simulink model "NDT_Localization"  (R2022a)
settings: Solver=FixedStepAuto  StartTime=0.0  StopTime=10.0  RelTol=1e-3
model workspace (MAT data in the model file):
  SL_ROS_VariableLengthArrays_MaxSizes : object (value not decoded)
undefined symbols (not defined in the file or in its folder): null
libraries: ros2lib x9, robotlib x8, simulink x1
(part 12 of 12)

== matlab function NDT_Localization/observation_callback/check_localizer/If Action Subsystem/register_measurement_impl/If Action Subsystem/If Action Subsystem/solve/If Action Subsystem1/For Iterator Subsystem/compute_next_step/If Action Subsystem1/psi_t/initial_objective_function/For Iterator Subsystem/gradient_jaco/gradient_col ==
  data: index input; gradient input; y output
function y = fcn(index,gradient)

y = gradient(:,index);

== matlab function NDT_Localization/observation_callback/check_localizer/If Action Subsystem/register_measurement_impl/If Action Subsystem/If Action Subsystem/solve/If Action Subsystem1/For Iterator Subsystem/compute_next_step/If Action Subsystem1/psi_t/initial_objective_function/For Iterator Subsystem/gradient_jaco/jaco_add ==
  data: jacobian input; jacobian output; index input; num input
function jacobian = fcn(jacobian,index,num)

jacobian(index) = jacobian(index)+num;

== matlab function NDT_Localization/observation_callback/check_localizer/If Action Subsystem/register_measurement_impl/If Action Subsystem/If Action Subsystem/solve/If Action Subsystem1/For Iterator Subsystem/compute_next_step/If Action Subsystem1/psi_t/initial_objective_function/angle_params/MATLAB Function ==
  data: x output; u input; y output; z output
function [x,y,z] = fcn(u)
x = u(3);
y = u(4);
z = u(5);

== matlab function NDT_Localization/observation_callback/check_localizer/If Action Subsystem/register_measurement_impl/If Action Subsystem/If Action Subsystem/solve/If Action Subsystem1/For Iterator Subsystem/compute_next_step/If Action Subsystem1/psi_t/initial_objective_function/gradient_angle/ga_a ==
  data: x input; out output; y input; z input
function out = fcn(x, y, z)
out = zeros(1,3); 
out(1) = x;
out(2) = y;
out(3) = z;

== matlab function NDT_Localization/observation_callback/check_localizer/If Action Subsystem/register_measurement_impl/If Action Subsystem/If Action Subsystem/solve/If Action Subsystem1/For Iterator Subsystem/compute_next_step/If Action Subsystem1/psi_t/initial_objective_function/gradient_angle/ga_b ==
  data: x input; out output; y input; z input
function out = fcn(x, y, z)
out = zeros(1,3); 
out(1) = x;
out(2) = y;
out(3) = z;

== matlab function NDT_Localization/observation_callback/check_localizer/If Action Subsystem/register_measurement_impl/If Action Subsystem/If Action Subsystem/solve/If Action Subsystem1/For Iterator Subsystem/compute_next_step/If Action Subsystem1/psi_t/initial_objective_function/gradient_angle/ga_c ==
  data: x input; out output; y input; z input
function out = fcn(x, y, z)
out = zeros(1,3); 
out(1) = x;
out(2) = y;
out(3) = z;

== matlab function NDT_Localization/observation_callback/check_localizer/If Action Subsystem/register_measurement_impl/If Action Subsystem/If Action Subsystem/solve/If Action Subsystem1/For Iterator Subsystem/compute_next_step/If Action Subsystem1/psi_t/initial_objective_function/gradient_angle/ga_d ==
  data: x input; out output; y input; z input
function out = fcn(x, y, z)
out = zeros(1,3); 
out(1) = x;
out(2) = y;
out(3) = z;

== matlab function NDT_Localization/observation_callback/check_localizer/If Action Subsystem/register_measurement_impl/If Action Subsystem/If Action Subsystem/solve/If Action Subsystem1/For Iterator Subsystem/compute_next_step/If Action Subsystem1/psi_t/initial_objective_function/gradient_angle/ga_e ==
  data: x input; out output; y input; z input
function out = fcn(x, y, z)
out = zeros(1,3); 
out(1) = x;
out(2) = y;
out(3) = z;

== matlab function NDT_Localization/observation_callback/check_localizer/If Action Subsystem/register_measurement_impl/If Action Subsystem/If Action Subsystem/solve/If Action Subsystem1/For Iterator Subsystem/compute_next_step/If Action Subsystem1/psi_t/initial_objective_function/gradient_angle/ga_f ==
  data: x input; out output; y input; z input
function out = fcn(x, y, z)
out = zeros(1,3); 
out(1) = x;
out(2) = y;
out(3) = z;

== matlab function NDT_Localization/observation_callback/check_localizer/If Action Subsystem/register_measurement_impl/If Action Subsystem/If Action Subsystem/solve/point_hessian ==
  data: hessian output; ha_a2 input; ha_a3 input; ha_b2 input; ha_b3 input; ha_c2 input; ha_c3 input; ha_d1 input; ha_d2 input; ha_d3 input; ha_e1 input; ha_e2 input; ha_e3 input; ha_f1 input; ha_f2 input; ha_f3 input
function hessian = fcn(ha_a2, ha_a3, ha_b2, ha_b3, ha_c2, ha_c3, ha_d1, ha_d2, ha_d3, ha_e1, ha_e2, ha_e3, ha_f1, ha_f2, ha_f3)

hessian = zeros(18,6,"single");
hessian(9,3) = [0.0 ha_a2 ha_a3];
hessian(12,3) = [0.0 ha_b2 ha_b3];
hessian(15,3) = [0.0 ha_c2 ha_c3];
hessian(9,4) = [0.0 ha_b2 ha_b3];
hessian(12,4) = [ha_d1 ha_d2 ha_d3];
hessian(15,4) = [ha_e1 ha_e2 ha_e3];
hessian(9,5) = [0.0 ha_c2 ha_c3];
hessian(12,5) = [ha_e1 ha_e2 ha_e3]:
hessian(15,5) = [ha_f1 ha_f2 ha_f3];

== matlab function NDT_Localization/observation_callback/check_localizer/If Action Subsystem/register_measurement_impl/If Action Subsystem/If Action Subsystem/solve/If Action Subsystem1/For Iterator Subsystem/compute_next_step/If Action Subsystem1/psi_t/initial_objective_function/gradient_angle/ga_g ==
  data: x input; out output; y input; z input
function out = fcn(x, y, z)
out = zeros(1,3); 
out(1) = x;
out(2) = y;
out(3) = z;

== matlab function NDT_Localization/observation_callback/check_localizer/If Action Subsystem/register_measurement_impl/If Action Subsystem/If Action Subsystem/solve/If Action Subsystem1/For Iterator Subsystem/compute_next_step/If Action Subsystem1/psi_t/initial_objective_function/gradient_angle/ga_h ==
  data: x input; out output; y input; z input
function out = fcn(x, y, z)
out = zeros(1,3); 
out(1) = x;
out(2) = y;
out(3) = z;

== matlab function NDT_Localization/observation_callback/check_localizer/If Action Subsystem/register_measurement_impl/If Action Subsystem/If Action Subsystem/solve/If Action Subsystem1/For Iterator Subsystem/compute_next_step/If Action Subsystem1/psi_t/initial_objective_function/point_gradient ==
  data: hessian output; ga_a input; ga_b input; ga_c input; ga_d input; ga_e input; ga_f input; ga_g input; ga_h input
function hessian = fcn(ga_a, ga_b, ga_c, ga_d, ga_e, ga_f, ga_g, ga_h)

hessian = zeros(3,6,"single");
hessian(1,3) = ga_a;
hessian(2,3) = ga_b;
hessian(0,4) = ga_c;
hessian(1,4) = ga_d;
hessian(2,4) = ga_e;
hessian(0,5) = ga_f;
hessian(1,5) = ga_g;
hessian(2,5) = ga_h;

== matlab function NDT_Localization/observation_callback/check_localizer/If Action Subsystem/register_measurement_impl/If Action Subsystem/If Action Subsystem/solve/If Action Subsystem1/For Iterator Subsystem/compute_next_step/If Action Subsystem1/psi_t/initial_objective_function/set_jacobian ==
  data: jacobian output
function jacobian = fcn()

jacobian = zeros(6,1,"single");

== matlab function NDT_Localization/observation_callback/check_localizer/If Action Subsystem/register_measurement_impl/If Action Subsystem/If Action Subsystem/solve/If Action Subsystem1/For Iterator Subsystem/compute_next_step/If Action Subsystem1/psi_t/objective_function/For Iterator Subsystem/Affine ==
  data: out output; u input
function out = fcn(u)

tform = affine3d;
pt = pointCloud(u);
xyz = pctransform(pt,tform);
out = xyz.Location;

== matlab function NDT_Localization/observation_callback/check_localizer/If Action Subsystem/register_measurement_impl/If Action Subsystem/If Action Subsystem/solve/If Action Subsystem1/For Iterator Subsystem/compute_next_step/If Action Subsystem1/psi_t/objective_function/For Iterator Subsystem/MATLAB Function ==
  data: data input; pt output; index input
function pt = fcn(data,index)

pt = data(index);

== matlab function NDT_Localization/observation_callback/check_localizer/If Action Subsystem/register_measurement_impl/If Action Subsystem/If Action Subsystem/solve/If Action Subsystem1/For Iterator Subsystem/compute_next_step/If Action Subsystem1/psi_t/objective_function/For Iterator Subsystem/gradient_jaco/gradient_col ==
  data: index input; gradient input; y output
function y = fcn(index,gradient)

y = gradient(:,index);

== matlab function NDT_Localization/observation_callback/check_localizer/If Action Subsystem/register_measurement_impl/If Action Subsystem/If Action Subsystem/solve/If Action Subsystem1/For Iterator Subsystem/compute_next_step/If Action Subsystem1/psi_t/objective_function/For Iterator Subsystem/gradient_jaco/jaco_add ==
  data: jacobian input; jacobian output; index input; num input
function jacobian = fcn(jacobian,index,num)

jacobian(index) = jacobian(index)+num;

== matlab function NDT_Localization/observation_callback/check_localizer/If Action Subsystem/register_measurement_impl/If Action Subsystem/If Action Subsystem/solve/If Action Subsystem1/For Iterator Subsystem/compute_next_step/If Action Subsystem1/psi_t/objective_function/angle_params/MATLAB Function ==
  data: x output; u input; y output; z output
function [x,y,z] = fcn(u)
x = u(3);
y = u(4);
z = u(5);

== matlab function NDT_Localization/observation_callback/check_localizer/If Action Subsystem/register_measurement_impl/If Action Subsystem/If Action Subsystem/solve/If Action Subsystem1/For Iterator Subsystem/compute_next_step/If Action Subsystem1/psi_t/objective_function/gradient_angle/ga_a ==
  data: x input; out output; y input; z input
function out = fcn(x, y, z)
out = zeros(1,3); 
out(1) = x;
out(2) = y;
out(3) = z;

== matlab function NDT_Localization/observation_callback/check_localizer/If Action Subsystem/register_measurement_impl/If Action Subsystem/If Action Subsystem/solve/If Action Subsystem1/For Iterator Subsystem/compute_next_step/If Action Subsystem1/psi_t/objective_function/gradient_angle/ga_b ==
  data: x input; out output; y input; z input
function out = fcn(x, y, z)
out = zeros(1,3); 
out(1) = x;
out(2) = y;
out(3) = z;

== matlab function NDT_Localization/observation_callback/check_localizer/If Action Subsystem/register_measurement_impl/If Action Subsystem/If Action Subsystem/solve/If Action Subsystem1/For Iterator Subsystem/compute_next_step/If Action Subsystem1/psi_t/objective_function/gradient_angle/ga_c ==
  data: x input; out output; y input; z input
function out = fcn(x, y, z)
out = zeros(1,3); 
out(1) = x;
out(2) = y;
out(3) = z;

== matlab function NDT_Localization/observation_callback/check_localizer/If Action Subsystem/register_measurement_impl/If Action Subsystem/If Action Subsystem/solve/If Action Subsystem1/For Iterator Subsystem/compute_next_step/If Action Subsystem1/psi_t/objective_function/gradient_angle/ga_d ==
  data: x input; out output; y input; z input
function out = fcn(x, y, z)
out = zeros(1,3); 
out(1) = x;
out(2) = y;
out(3) = z;

== matlab function NDT_Localization/observation_callback/check_localizer/If Action Subsystem/register_measurement_impl/If Action Subsystem/If Action Subsystem/solve/If Action Subsystem1/For Iterator Subsystem/compute_next_step/If Action Subsystem1/psi_t/objective_function/gradient_angle/ga_e ==
  data: x input; out output; y input; z input
function out = fcn(x, y, z)
out = zeros(1,3); 
out(1) = x;
out(2) = y;
out(3) = z;

== matlab function NDT_Localization/observation_callback/check_localizer/If Action Subsystem/register_measurement_impl/If Action Subsystem/If Action Subsystem/solve/If Action Subsystem1/For Iterator Subsystem/compute_next_step/If Action Subsystem1/psi_t/objective_function/gradient_angle/ga_f ==
  data: x input; out output; y input; z input
function out = fcn(x, y, z)
out = zeros(1,3); 
out(1) = x;
out(2) = y;
out(3) = z;

== matlab function NDT_Localization/observation_callback/check_localizer/If Action Subsystem/register_measurement_impl/If Action Subsystem/If Action Subsystem/solve/If Action Subsystem1/For Iterator Subsystem/compute_next_step/If Action Subsystem1/psi_t/objective_function/gradient_angle/ga_g ==
  data: x input; out output; y input; z input
function out = fcn(x, y, z)
out = zeros(1,3); 
out(1) = x;
out(2) = y;
out(3) = z;

== matlab function NDT_Localization/observation_callback/check_localizer/If Action Subsystem/register_measurement_impl/If Action Subsystem/If Action Subsystem/solve/If Action Subsystem1/For Iterator Subsystem/compute_next_step/If Action Subsystem1/psi_t/objective_function/gradient_angle/ga_h ==
  data: x input; out output; y input; z input
function out = fcn(x, y, z)
out = zeros(1,3); 
out(1) = x;
out(2) = y;
out(3) = z;

== matlab function NDT_Localization/observation_callback/check_localizer/If Action Subsystem/register_measurement_impl/If Action Subsystem/If Action Subsystem/solve/If Action Subsystem1/For Iterator Subsystem/compute_next_step/If Action Subsystem1/psi_t/objective_function/point_gradient ==
  data: hessian output; ga_a input; ga_b input; ga_c input; ga_d input; ga_e input; ga_f input; ga_g input; ga_h input
function hessian = fcn(ga_a, ga_b, ga_c, ga_d, ga_e, ga_f, ga_g, ga_h)

hessian = zeros(3,6,"single");
hessian(1,3) = ga_a;
hessian(2,3) = ga_b;
hessian(0,4) = ga_c;
hessian(1,4) = ga_d;
hessian(2,4) = ga_e;
hessian(0,5) = ga_f;
hessian(1,5) = ga_g;
hessian(2,5) = ga_h;

== matlab function NDT_Localization/observation_callback/check_localizer/If Action Subsystem/register_measurement_impl/If Action Subsystem/If Action Subsystem/solve/If Action Subsystem1/For Iterator Subsystem/compute_next_step/If Action Subsystem1/psi_t/objective_function/set_jacobian ==
  data: jacobian output
function jacobian = fcn()

jacobian = zeros(6,1,"single");

== matlab function NDT_Localization/observation_callback/check_localizer/If Action Subsystem/register_measurement_impl/If Action Subsystem/If Action Subsystem/solve/For Iterator Subsystem/For Iterator Subsystem/MATLAB Function1 ==
  data: index_i input; y output; index_j input; point_hessian input
function y = fcn(index_i,index_j,point_hessian)

y = point_hessian(3*index_i-2:3*index_i,index_j);

== matlab function NDT_Localization/observation_callback/check_localizer/If Action Subsystem/register_measurement_impl/If Action Subsystem/If Action Subsystem/solve/angle_params/MATLAB Function ==
  data: x output; u input; y output; z output
function [x,y,z] = fcn(u)
x = u(3);
y = u(4);
z = u(5);

== matlab function NDT_Localization/observation_callback/check_localizer/If Action Subsystem/register_measurement_impl/If Action Subsystem/If Action Subsystem/solve/gradient_angle/ga_a ==
  data: x input; out output; y input; z input
function out = fcn(x, y, z)
out = zeros(1,3); 
out(1) = x;
out(2) = y;
out(3) = z;

== matlab function NDT_Localization/observation_callback/check_localizer/If Action Subsystem/register_measurement_impl/If Action Subsystem/If Action Subsystem/solve/gradient_angle/ga_b ==
  data: x input; out output; y input; z input
function out = fcn(x, y, z)
out = zeros(1,3); 
out(1) = x;
out(2) = y;
out(3) = z;

== matlab function NDT_Localization/observation_callback/check_localizer/If Action Subsystem/register_measurement_impl/If Action Subsystem/If Action Subsystem/solve/gradient_angle/ga_c ==
  data: x input; out output; y input; z input
function out = fcn(x, y, z)
out = zeros(1,3); 
out(1) = x;
out(2) = y;
out(3) = z;

== matlab function NDT_Localization/observation_callback/check_localizer/If Action Subsystem/register_measurement_impl/If Action Subsystem/If Action Subsystem/solve/gradient_angle/ga_d ==
  data: x input; out output; y input; z input
function out = fcn(x, y, z)
out = zeros(1,3); 
out(1) = x;
out(2) = y;
out(3) = z;

== matlab function NDT_Localization/observation_callback/check_localizer/If Action Subsystem/register_measurement_impl/If Action Subsystem/If Action Subsystem/solve/gradient_angle/ga_e ==
  data: x input; out output; y input; z input
function out = fcn(x, y, z)
out = zeros(1,3); 
out(1) = x;
out(2) = y;
out(3) = z;

== matlab function NDT_Localization/observation_callback/check_localizer/If Action Subsystem/register_measurement_impl/If Action Subsystem/If Action Subsystem/solve/gradient_angle/ga_f ==
  data: x input; out output; y input; z input
function out = fcn(x, y, z)
out = zeros(1,3); 
out(1) = x;
out(2) = y;
out(3) = z;

== matlab function NDT_Localization/observation_callback/check_localizer/If Action Subsystem/register_measurement_impl/If Action Subsystem/If Action Subsystem/solve/gradient_angle/ga_g ==
  data: x input; out output; y input; z input
function out = fcn(x, y, z)
out = zeros(1,3); 
out(1) = x;
out(2) = y;
out(3) = z;

== matlab function NDT_Localization/observation_callback/check_localizer/If Action Subsystem/register_measurement_impl/If Action Subsystem/If Action Subsystem/solve/gradient_angle/ga_h ==
  data: x input; out output; y input; z input
function out = fcn(x, y, z)
out = zeros(1,3); 
out(1) = x;
out(2) = y;
out(3) = z;

== matlab function NDT_Localization/map_callback/check_localizer/set_map/set_map_impl/insert/insert_/If Action Subsystem/While Iterator Subsystem/MATLAB Function ==
  data: msg input; point output; id input
function point = fcn(msg, id)

point = msg(id);

== matlab function NDT_Localization/observation_callback/check_localizer/If Action Subsystem/register_measurement_impl/If Action Subsystem/If Action Subsystem/solve/hessian_angle/ha_a2 ==
  data: x input; out output; y input; z input
function out = fcn(x, y, z)
out = zeros(1,3); 
out(1) = x;
out(2) = y;
out(3) = z;

== matlab function NDT_Localization/observation_callback/check_localizer/If Action Subsystem/register_measurement_impl/If Action Subsystem/If Action Subsystem/solve/hessian_angle/ha_a3 ==
  data: x input; out output; y input; z input
function out = fcn(x, y, z)
out = zeros(1,3); 
out(1) = x;
out(2) = y;
out(3) = z;

== matlab function NDT_Localization/observation_callback/check_localizer/If Action Subsystem/register_measurement_impl/If Action Subsystem/If Action Subsystem/solve/hessian_angle/ha_b2 ==
  data: x input; out output; y input; z input
function out = fcn(x, y, z)
out = zeros(1,3); 
out(1) = x;
out(2) = y;
out(3) = z;

== matlab function NDT_Localization/observation_callback/check_localizer/If Action Subsystem/register_measurement_impl/If Action Subsystem/If Action Subsystem/solve/hessian_angle/ha_b3 ==
  data: x input; out output; y input; z input
function out = fcn(x, y, z)
out = zeros(1,3); 
out(1) = x;
out(2) = y;
out(3) = z;

== matlab function NDT_Localization/observation_callback/check_localizer/If Action Subsystem/register_measurement_impl/If Action Subsystem/If Action Subsystem/solve/hessian_angle/ha_c2 ==
  data: x input; out output; y input; z input
function out = fcn(x, y, z)
out = zeros(1,3); 
out(1) = x;
out(2) = y;
out(3) = z;

== matlab function NDT_Localization/observation_callback/check_localizer/If Action Subsystem/register_measurement_impl/If Action Subsystem/If Action Subsystem/solve/hessian_angle/ha_c3 ==
  data: x input; out output; y input; z input
function out = fcn(x, y, z)
out = zeros(1,3); 
out(1) = x;
out(2) = y;
out(3) = z;

== matlab function NDT_Localization/observation_callback/check_localizer/If Action Subsystem/register_measurement_impl/If Action Subsystem/If Action Subsystem/solve/hessian_angle/ha_d1 ==
  data: x input; out output; y input; z input
function out = fcn(x, y, z)
out = zeros(1,3); 
out(1) = x;
out(2) = y;
out(3) = z;

== matlab function NDT_Localization/observation_callback/check_localizer/If Action Subsystem/register_measurement_impl/If Action Subsystem/If Action Subsystem/solve/hessian_angle/ha_d2 ==
  data: x input; out output; y input; z input
function out = fcn(x, y, z)
out = zeros(1,3); 
out(1) = x;
out(2) = y;
out(3) = z;

== matlab function NDT_Localization/observation_callback/check_localizer/If Action Subsystem/register_measurement_impl/If Action Subsystem/If Action Subsystem/solve/hessian_angle/ha_d3 ==
  data: x input; out output; y input; z input
function out = fcn(x, y, z)
out = zeros(1,3); 
out(1) = x;
out(2) = y;
out(3) = z;

== matlab function NDT_Localization/map_callback/check_localizer/set_map/set_map_impl/insert/insert_/validate_pcl_map/check_fields/check_fields_name/MATLAB Function ==
  data: names output; data input; data1 input; data2 input; data3 input; data4 input; data5 input; data6 input; data7 input; data8 input; data9 input
function names = fcn(data, data1, data2, data3, data4, data5, data6, data7, data8, data9)

names = [data data1 data2 data3 data4 data5 data6 data7 data8 data9];

== matlab function NDT_Localization/observation_callback/check_localizer/If Action Subsystem/register_measurement_impl/If Action Subsystem/If Action Subsystem/solve/hessian_angle/ha_e1 ==
  data: x input; out output; y input; z input
function out = fcn(x, y, z)
out = zeros(1,3); 
out(1) = x;
out(2) = y;
out(3) = z;

== matlab function NDT_Localization/observation_callback/check_localizer/If Action Subsystem/register_measurement_impl/If Action Subsystem/If Action Subsystem/solve/hessian_angle/ha_e2 ==
  data: x input; out output; y input; z input
function out = fcn(x, y, z)
out = zeros(1,3); 
out(1) = x;
out(2) = y;
out(3) = z;

== matlab function NDT_Localization/observation_callback/check_localizer/If Action Subsystem/register_measurement_impl/If Action Subsystem/If Action Subsystem/solve/hessian_angle/ha_e3 ==
  data: x input; out output; y input; z input
function out = fcn(x, y, z)
out = zeros(1,3); 
out(1) = x;
out(2) = y;
out(3) = z;

== matlab function NDT_Localization/observation_callback/check_localizer/If Action Subsystem/register_measurement_impl/If Action Subsystem/If Action Subsystem/solve/hessian_angle/ha_f1 ==
  data: x input; out output; y input; z input
function out = fcn(x, y, z)
out = zeros(1,3); 
out(1) = x;
out(2) = y;
out(3) = z;

== matlab function NDT_Localization/observation_callback/check_localizer/If Action Subsystem/register_measurement_impl/If Action Subsystem/If Action Subsystem/solve/hessian_angle/ha_f2 ==
  data: x input; out output; y input; z input
function out = fcn(x, y, z)
out = zeros(1,3); 
out(1) = x;
out(2) = y;
out(3) = z;

== matlab function NDT_Localization/observation_callback/check_localizer/If Action Subsystem/register_measurement_impl/If Action Subsystem/If Action Subsystem/solve/hessian_angle/ha_f3 ==
  data: x input; out output; y input; z input
function out = fcn(x, y, z)
out = zeros(1,3); 
out(1) = x;
out(2) = y;
out(3) = z;

== matlab function NDT_Localization/observation_callback/check_localizer/If Action Subsystem/register_measurement_impl/If Action Subsystem/If Action Subsystem/solve/If Action Subsystem1/For Iterator Subsystem/MATLAB Function ==
  data: jacobian input; opt_direction output; hessian input
function opt_direction = fcn(jacobian, hessian)

opt_direction = hessian\jacobian;

== matlab function NDT_Localization/observation_callback/check_localizer/If Action Subsystem/register_measurement_impl/If Action Subsystem/If Action Subsystem/solve/If Action Subsystem1/For Iterator Subsystem/Allfinite_score ==
  data: u input; y output
function y = fcn(u)

y = allfinite(u);

== matlab function NDT_Localization/observation_callback/check_localizer/If Action Subsystem/register_measurement_impl/If Action Subsystem/If Action Subsystem/solve/If Action Subsystem1/For Iterator Subsystem/Allfinite_jacobian ==
  data: u input; y output
function y = fcn(u)

y = allfinite(u);

== matlab function NDT_Localization/observation_callback/check_localizer/If Action Subsystem/register_measurement_impl/If Action Subsystem/If Action Subsystem/solve/If Action Subsystem1/For Iterator Subsystem/Allfinite_hessian ==
  data: u input; y output
function y = fcn(u)

y = allfinite(u);

== matlab function NDT_Localization/observation_callback/check_localizer/If Action Subsystem/register_measurement_impl/If Action Subsystem/If Action Subsystem/solve/If Action Subsystem1/For Iterator Subsystem/Allfinite_direction ==
  data: u input; y output
function y = fcn(u)

y = allfinite(u);

== matlab function NDT_Localization/observation_callback/check_localizer/If Action Subsystem/register_measurement_impl/If Action Subsystem/If Action Subsystem/solve/If Action Subsystem1/For Iterator Subsystem/For Iterator Subsystem/For Iterator Subsystem/MATLAB Function ==
  data: u input; y output
function y = fcn(u)

y = size(u,2);

== matlab function NDT_Localization/observation_callback/check_localizer/If Action Subsystem/register_measurement_impl/If Action Subsystem/If Action Subsystem/solve/If Action Subsystem1/For Iterator Subsystem/For Iterator Subsystem/For Iterator Subsystem/MATLAB Function1 ==
  data: index_i input; y output; index_j input; point_hessian input
function y = fcn(index_i,index_j,point_hessian)

y = point_hessian(3*index_i-2:3*index_i,index_j);

== matlab function NDT_Localization/observation_callback/check_localizer/If Action Subsystem/register_measurement_impl/If Action Subsystem/If Action Subsystem/solve/If Action Subsystem1/For Iterator Subsystem/For Iterator Subsystem/For Iterator Subsystem/gradient_col_i ==
  data: index_i input; gradient input; y output
function y = fcn(index_i,gradient)

y = gradient(:,index_i);

== matlab function NDT_Localization/observation_callback/check_localizer/If Action Subsystem/register_measurement_impl/If Action Subsystem/If Action Subsystem/solve/If Action Subsystem1/For Iterator Subsystem/For Iterator Subsystem/For Iterator Subsystem/gradient_col_j ==
  data: index_j input; gradient input; y output
function y = fcn(index_j,gradient)

y = gradient(:,index_j);

== matlab function NDT_Localization/observation_callback/check_localizer/If Action Subsystem/register_measurement_impl/If Action Subsystem/If Action Subsystem/solve/If Action Subsystem1/For Iterator Subsystem/For Iterator Subsystem/For Iterator Subsystem/hessian_add ==
  data: hessian input; hessian output; index_i input; index_j input; num input
function hessian = fcn(hessian,index_i,index_j,num)

hessian(index_i,index_j) = hessian(index_i,index_j)+num;

== matlab function NDT_Localization/observation_callback/check_localizer/If Action Subsystem/register_measurement_impl/If Action Subsystem/If Action Subsystem/solve/If Action Subsystem1/For Iterator Subsystem/For Iterator Subsystem/MATLAB Function ==
  data: data input; pt output; index input
function pt = fcn(data,index)

pt = data(index);

== matlab function NDT_Localization/observation_callback/check_localizer/If Action Subsystem/register_measurement_impl/If Action Subsystem/If Action Subsystem/solve/If Action Subsystem1/For Iterator Subsystem/For Iterator Subsystem/gradient_jaco/gradient_col ==
  data: index input; gradient input; y output
function y = fcn(index,gradient)

y = gradient(:,index);

== matlab function NDT_Localization/observation_callback/check_localizer/If Action Subsystem/register_measurement_impl/If Action Subsystem/If Action Subsystem/solve/If Action Subsystem1/For Iterator Subsystem/For Iterator Subsystem/gradient_jaco/jaco_add ==
  data: jacobian input; jacobian output; index input; num input
function jacobian = fcn(jacobian,index,num)

jacobian(index) = jacobian(index)+num;

== matlab function NDT_Localization/map_callback/check_localizer/set_map/set_map_impl/insert/insert_/validate_pcl_map/check_fields/check_fields_name/For Iterator Subsystem1/MATLAB Function ==
  data: index input; name input string; name_o output string; data input string; fields output string
function [name_o, fields] = fcn(index, name, data)

name_o = name(index);
fields = data(index);

== matlab function NDT_Localization/observation_callback/check_localizer/If Action Subsystem/register_measurement_impl/If Action Subsystem/If Action Subsystem/solve/If Action Subsystem1/For Iterator Subsystem/angle_params/MATLAB Function ==
  data: x output; u input; y output; z output
function [x,y,z] = fcn(u)
x = u(3);
y = u(4);
z = u(5);

== matlab function NDT_Localization/observation_callback/check_localizer/If Action Subsystem/register_measurement_impl/If Action Subsystem/If Action Subsystem/solve/If Action Subsystem1/For Iterator Subsystem/gradient_angle/ga_a ==
  data: x input; out output; y input; z input
function out = fcn(x, y, z)
out = zeros(1,3); 
out(1) = x;
out(2) = y;
out(3) = z;

== matlab function NDT_Localization/observation_callback/check_localizer/If Action Subsystem/register_measurement_impl/If Action Subsystem/If Action Subsystem/solve/If Action Subsystem1/For Iterator Subsystem/gradient_angle/ga_b ==
  data: x input; out output; y input; z input
function out = fcn(x, y, z)
out = zeros(1,3); 
out(1) = x;
out(2) = y;
out(3) = z;

== matlab function NDT_Localization/observation_callback/check_localizer/If Action Subsystem/register_measurement_impl/If Action Subsystem/If Action Subsystem/solve/If Action Subsystem1/For Iterator Subsystem/gradient_angle/ga_c ==
  data: x input; out output; y input; z input
function out = fcn(x, y, z)
out = zeros(1,3); 
out(1) = x;
out(2) = y;
out(3) = z;

== matlab function NDT_Localization/observation_callback/check_localizer/If Action Subsystem/register_measurement_impl/If Action Subsystem/If Action Subsystem/solve/If Action Subsystem1/For Iterator Subsystem/gradient_angle/ga_d ==
  data: x input; out output; y input; z input
function out = fcn(x, y, z)
out = zeros(1,3); 
out(1) = x;
out(2) = y;
out(3) = z;

== matlab function NDT_Localization/observation_callback/check_localizer/If Action Subsystem/register_measurement_impl/If Action Subsystem/If Action Subsystem/solve/If Action Subsystem1/For Iterator Subsystem/gradient_angle/ga_e ==
  data: x input; out output; y input; z input
function out = fcn(x, y, z)
out = zeros(1,3); 
out(1) = x;
out(2) = y;
out(3) = z;

== matlab function NDT_Localization/observation_callback/check_localizer/If Action Subsystem/register_measurement_impl/If Action Subsystem/If Action Subsystem/solve/If Action Subsystem1/For Iterator Subsystem/gradient_angle/ga_f ==
  data: x input; out output; y input; z input
function out = fcn(x, y, z)
out = zeros(1,3); 
out(1) = x;
out(2) = y;
out(3) = z;

== matlab function NDT_Localization/observation_callback/check_localizer/If Action Subsystem/register_measurement_impl/If Action Subsystem/If Action Subsystem/solve/If Action Subsystem1/For Iterator Subsystem/gradient_angle/ga_g ==
  data: x input; out output; y input; z input
function out = fcn(x, y, z)
out = zeros(1,3); 
out(1) = x;
out(2) = y;
out(3) = z;

== matlab function NDT_Localization/observation_callback/check_localizer/If Action Subsystem/register_measurement_impl/If Action Subsystem/If Action Subsystem/solve/If Action Subsystem1/For Iterator Subsystem/gradient_angle/ga_h ==
  data: x input; out output; y input; z input
function out = fcn(x, y, z)
out = zeros(1,3); 
out(1) = x;
out(2) = y;
out(3) = z;

== matlab function NDT_Localization/observation_callback/check_localizer/If Action Subsystem/register_measurement_impl/If Action Subsystem/If Action Subsystem/solve/If Action Subsystem1/For Iterator Subsystem/hessian_angle/ha_a2 ==
  data: x input; out output; y input; z input
function out = fcn(x, y, z)
out = zeros(1,3); 
out(1) = x;
out(2) = y;
out(3) = z;

== matlab function NDT_Localization/observation_callback/check_localizer/If Action Subsystem/register_measurement_impl/If Action Subsystem/If Action Subsystem/solve/If Action Subsystem1/For Iterator Subsystem/hessian_angle/ha_a3 ==
  data: x input; out output; y input; z input
function out = fcn(x, y, z)
out = zeros(1,3); 
out(1) = x;
out(2) = y;
out(3) = z;

== matlab function NDT_Localization/observation_callback/check_localizer/If Action Subsystem/register_measurement_impl/If Action Subsystem/If Action Subsystem/solve/If Action Subsystem1/For Iterator Subsystem/hessian_angle/ha_b2 ==
  data: x input; out output; y input; z input
function out = fcn(x, y, z)
out = zeros(1,3); 
out(1) = x;
out(2) = y;
out(3) = z;

== matlab function NDT_Localization/map_callback/check_localizer/set_map/set_map_impl/insert/insert_/If Action Subsystem/While Iterator Subsystem/MATLAB Function1 ==
  data: point input; point_step input; xx output; offset input; xy output; xz output; yy output; yz output; zz output
function [xx,xy,xz,yy,yz,zz] = fcn(point, point_step, offset)

xx = point(offset(4):offset(4)+point_step-1);
xy = point(offset(5):offset(5)+point_step-1);
xz = point(offset(6):offset(6)+point_step-1);
yy = point(offset(7):offset(7)+point_step-1);
yz = point(offset(8):offset(8)+point_step-1);
zz = point(offset(9):offset(9)+point_step-1);

== matlab function NDT_Localization/observation_callback/check_localizer/If Action Subsystem/register_measurement_impl/If Action Subsystem/If Action Subsystem/solve/If Action Subsystem1/For Iterator Subsystem/hessian_angle/ha_b3 ==
  data: x input; out output; y input; z input
function out = fcn(x, y, z)
out = zeros(1,3); 
out(1) = x;
out(2) = y;
out(3) = z;

== matlab function NDT_Localization/observation_callback/check_localizer/If Action Subsystem/register_measurement_impl/If Action Subsystem/If Action Subsystem/solve/If Action Subsystem1/For Iterator Subsystem/hessian_angle/ha_c2 ==
  data: x input; out output; y input; z input
function out = fcn(x, y, z)
out = zeros(1,3); 
out(1) = x;
out(2) = y;
out(3) = z;

== matlab function NDT_Localization/observation_callback/check_localizer/If Action Subsystem/register_measurement_impl/If Action Subsystem/If Action Subsystem/solve/If Action Subsystem1/For Iterator Subsystem/hessian_angle/ha_c3 ==
  data: x input; out output; y input; z input
function out = fcn(x, y, z)
out = zeros(1,3); 
out(1) = x;
out(2) = y;
out(3) = z;

== matlab function NDT_Localization/observation_callback/check_localizer/If Action Subsystem/register_measurement_impl/If Action Subsystem/If Action Subsystem/solve/If Action Subsystem1/For Iterator Subsystem/hessian_angle/ha_d1 ==
  data: x input; out output; y input; z input
function out = fcn(x, y, z)
out = zeros(1,3); 
out(1) = x;
out(2) = y;
out(3) = z;

== matlab function NDT_Localization/observation_callback/check_localizer/If Action Subsystem/register_measurement_impl/If Action Subsystem/If Action Subsystem/solve/If Action Subsystem1/For Iterator Subsystem/hessian_angle/ha_d2 ==
  data: x input; out output; y input; z input
function out = fcn(x, y, z)
out = zeros(1,3); 
out(1) = x;
out(2) = y;
out(3) = z;

== matlab function NDT_Localization/observation_callback/check_localizer/If Action Subsystem/register_measurement_impl/If Action Subsystem/If Action Subsystem/solve/If Action Subsystem1/For Iterator Subsystem/hessian_angle/ha_d3 ==
  data: x input; out output; y input; z input
function out = fcn(x, y, z)
out = zeros(1,3); 
out(1) = x;
out(2) = y;
out(3) = z;

== matlab function NDT_Localization/observation_callback/check_localizer/If Action Subsystem/register_measurement_impl/If Action Subsystem/If Action Subsystem/solve/If Action Subsystem1/For Iterator Subsystem/hessian_angle/ha_e1 ==
  data: x input; out output; y input; z input
function out = fcn(x, y, z)
out = zeros(1,3); 
out(1) = x;
out(2) = y;
out(3) = z;

== matlab function NDT_Localization/observation_callback/check_localizer/If Action Subsystem/register_measurement_impl/If Action Subsystem/If Action Subsystem/solve/If Action Subsystem1/For Iterator Subsystem/hessian_angle/ha_e2 ==
  data: x input; out output; y input; z input
function out = fcn(x, y, z)
out = zeros(1,3); 
out(1) = x;
out(2) = y;
out(3) = z;

== matlab function NDT_Localization/observation_callback/check_localizer/If Action Subsystem/register_measurement_impl/If Action Subsystem/If Action Subsystem/solve/If Action Subsystem1/For Iterator Subsystem/hessian_angle/ha_e3 ==
  data: x input; out output; y input; z input
function out = fcn(x, y, z)
out = zeros(1,3); 
out(1) = x;
out(2) = y;
out(3) = z;

== matlab function NDT_Localization/observation_callback/check_localizer/If Action Subsystem/register_measurement_impl/If Action Subsystem/If Action Subsystem/solve/If Action Subsystem1/For Iterator Subsystem/hessian_angle/ha_f1 ==
  data: x input; out output; y input; z input
function out = fcn(x, y, z)
out = zeros(1,3); 
out(1) = x;
out(2) = y;
out(3) = z;

== matlab function NDT_Localization/observation_callback/check_localizer/If Action Subsystem/register_measurement_impl/If Action Subsystem/If Action Subsystem/solve/If Action Subsystem1/For Iterator Subsystem/hessian_angle/ha_f2 ==
  data: x input; out output; y input; z input
function out = fcn(x, y, z)
out = zeros(1,3); 
out(1) = x;
out(2) = y;
out(3) = z;

== matlab function NDT_Localization/observation_callback/check_localizer/If Action Subsystem/register_measurement_impl/If Action Subsystem/If Action Subsystem/solve/If Action Subsystem1/For Iterator Subsystem/hessian_angle/ha_f3 ==
  data: x input; out output; y input; z input
function out = fcn(x, y, z)
out = zeros(1,3); 
out(1) = x;
out(2) = y;
out(3) = z;

== matlab function NDT_Localization/observation_callback/check_localizer/If Action Subsystem/register_measurement_impl/If Action Subsystem/If Action Subsystem/solve/If Action Subsystem1/For Iterator Subsystem/point_gradient ==
  data: hessian output; ga_a input; ga_b input; ga_c input; ga_d input; ga_e input; ga_f input; ga_g input; ga_h input
function hessian = fcn(ga_a, ga_b, ga_c, ga_d, ga_e, ga_f, ga_g, ga_h)

hessian = zeros(3,6,"single");
hessian(1,3) = ga_a;
hessian(2,3) = ga_b;
hessian(0,4) = ga_c;
hessian(1,4) = ga_d;
hessian(2,4) = ga_e;
hessian(0,5) = ga_f;
hessian(1,5) = ga_g;
hessian(2,5) = ga_h;

== matlab function NDT_Localization/observation_callback/check_localizer/If Action Subsystem/register_measurement_impl/If Action Subsystem/If Action Subsystem/solve/If Action Subsystem1/For Iterator Subsystem/point_hessian ==
  data: hessian output; ha_a2 input; ha_a3 input; ha_b2 input; ha_b3 input; ha_c2 input; ha_c3 input; ha_d1 input; ha_d2 input; ha_d3 input; ha_e1 input; ha_e2 input; ha_e3 input; ha_f1 input; ha_f2 input; ha_f3 input
function hessian = fcn(ha_a2, ha_a3, ha_b2, ha_b3, ha_c2, ha_c3, ha_d1, ha_d2, ha_d3, ha_e1, ha_e2, ha_e3, ha_f1, ha_f2, ha_f3)

hessian = zeros(18,6,"single");
hessian(9,3) = [0.0 ha_a2 ha_a3];
hessian(12,3) = [0.0 ha_b2 ha_b3];
hessian(15,3) = [0.0 ha_c2 ha_c3];
hessian(9,4) = [0.0 ha_b2 ha_b3];
hessian(12,4) = [ha_d1 ha_d2 ha_d3];
hessian(15,4) = [ha_e1 ha_e2 ha_e3];
hessian(9,5) = [0.0 ha_c2 ha_c3];
hessian(12,5) = [ha_e1 ha_e2 ha_e3]:
hessian(15,5) = [ha_f1 ha_f2 ha_f3];

== matlab function NDT_Localization/map_callback/check_localizer/set_map/set_map_impl/insert/insert_/If Action Subsystem/While Iterator Subsystem/MATLAB Function2 ==
  data: xx input; inv_covariance output; xy input; xz input; yy input; yz input; zz input
function inv_covariance = fcn(xx,xy,xz,yy,yz,zz)

inv_covariance = [xx xy xz; xy yy yz; xz yz zz;];

== matlab function NDT_Localization/observation_callback/check_localizer/If Action Subsystem/register_measurement_impl/If Action Subsystem/If Action Subsystem/solve/If Action Subsystem1/For Iterator Subsystem/set_hessian ==
  data: hessian output
function hessian = fcn()

hessian = zeros(6,6,"single");

== matlab function NDT_Localization/observation_callback/check_localizer/If Action Subsystem/register_measurement_impl/If Action Subsystem/If Action Subsystem/solve/If Action Subsystem1/For Iterator Subsystem/set_jacobian ==
  data: jacobian output
function jacobian = fcn()

jacobian = zeros(6,1,"single");

== matlab function NDT_Localization/observation_callback/check_localizer/If Action Subsystem/register_measurement_impl/If Action Subsystem/If Action Subsystem/solve/If Action Subsystem1/For Iterator Subsystem/compute_next_step/If Action Subsystem1/For Iterator Subsystem/If Action Subsystem/If Action Subsystem3/phi_t/For Iterator Subsystem/Affine ==
  data: out output; u input
function out = fcn(u)

tform = affine3d;
pt = pointCloud(u);
xyz = pctransform(pt,tform);
out = xyz.Location;

== matlab function NDT_Localization/observation_callback/check_localizer/If Action Subsystem/register_measurement_impl/If Action Subsystem/If Action Subsystem/solve/If Action Subsystem1/For Iterator Subsystem/compute_next_step/If Action Subsystem1/For Iterator Subsystem/If Action Subsystem/If Action Subsystem3/phi_t/For Iterator Subsystem/MATLAB Function ==
  data: data input; pt output; index input
function pt = fcn(data,index)

pt = data(index);

== matlab function NDT_Localization/observation_callback/check_localizer/If Action Subsystem/register_measurement_impl/If Action Subsystem/If Action Subsystem/solve/If Action Subsystem1/For Iterator Subsystem/compute_next_step/If Action Subsystem1/For Iterator Subsystem/If Action Subsystem/If Action Subsystem3/phi_t/For Iterator Subsystem/gradient_jaco/gradient_col ==
  data: index input; gradient input; y output
function y = fcn(index,gradient)

y = gradient(:,index);

== matlab function NDT_Localization/observation_callback/check_localizer/If Action Subsystem/register_measurement_impl/If Action Subsystem/If Action Subsystem/solve/If Action Subsystem1/For Iterator Subsystem/compute_next_step/If Action Subsystem1/For Iterator Subsystem/If Action Subsystem/If Action Subsystem3/phi_t/For Iterator Subsystem/gradient_jaco/jaco_add ==
  data: jacobian input; jacobian output; index input; num input
function jacobian = fcn(jacobian,index,num)

jacobian(index) = jacobian(index)+num;

== matlab function NDT_Localization/observation_callback/check_localizer/If Action Subsystem/register_measurement_impl/If Action Subsystem/If Action Subsystem/solve/If Action Subsystem1/For Iterator Subsystem/compute_next_step/If Action Subsystem1/For Iterator Subsystem/If Action Subsystem/If Action Subsystem3/phi_t/angle_params/MATLAB Function ==
  data: x output; u input; y output; z output
function [x,y,z] = fcn(u)
x = u(3);
y = u(4);
z = u(5);

== matlab function NDT_Localization/observation_callback/check_localizer/If Action Subsystem/register_measurement_impl/If Action Subsystem/If Action Subsystem/solve/If Action Subsystem1/For Iterator Subsystem/compute_next_step/If Action Subsystem1/For Iterator Subsystem/If Action Subsystem/If Action Subsystem3/phi_t/gradient_angle/ga_a ==
  data: x input; out output; y input; z input
function out = fcn(x, y, z)
out = zeros(1,3); 
out(1) = x;
out(2) = y;
out(3) = z;

== matlab function NDT_Localization/observation_callback/check_localizer/If Action Subsystem/register_measurement_impl/If Action Subsystem/If Action Subsystem/solve/If Action Subsystem1/For Iterator Subsystem/compute_next_step/If Action Subsystem1/For Iterator Subsystem/If Action Subsystem/If Action Subsystem3/phi_t/gradient_angle/ga_b ==
  data: x input; out output; y input; z input
function out = fcn(x, y, z)
out = zeros(1,3); 
out(1) = x;
out(2) = y;
out(3) = z;

== matlab function NDT_Localization/observation_callback/check_localizer/If Action Subsystem/register_measurement_impl/If Action Subsystem/If Action Subsystem/solve/If Action Subsystem1/For Iterator Subsystem/compute_next_step/If Action Subsystem1/For Iterator Subsystem/If Action Subsystem/If Action Subsystem3/phi_t/gradient_angle/ga_c ==
  data: x input; out output; y input; z input
function out = fcn(x, y, z)
out = zeros(1,3); 
out(1) = x;
out(2) = y;
out(3) = z;

== matlab function NDT_Localization/observation_callback/check_localizer/If Action Subsystem/register_measurement_impl/If Action Subsystem/If Action Subsystem/solve/If Action Subsystem1/For Iterator Subsystem/compute_next_step/If Action Subsystem1/For Iterator Subsystem/If Action Subsystem/If Action Subsystem3/phi_t/gradient_angle/ga_d ==
  data: x input; out output; y input; z input
function out = fcn(x, y, z)
out = zeros(1,3); 
out(1) = x;
out(2) = y;
out(3) = z;

== matlab function NDT_Localization/observation_callback/check_localizer/If Action Subsystem/register_measurement_impl/If Action Subsystem/If Action Subsystem/solve/If Action Subsystem1/For Iterator Subsystem/compute_next_step/If Action Subsystem1/For Iterator Subsystem/If Action Subsystem/If Action Subsystem3/phi_t/gradient_angle/ga_e ==
  data: x input; out output; y input; z input
function out = fcn(x, y, z)
out = zeros(1,3); 
out(1) = x;
out(2) = y;
out(3) = z;

== matlab function NDT_Localization/observation_callback/check_localizer/If Action Subsystem/register_measurement_impl/If Action Subsystem/If Action Subsystem/solve/If Action Subsystem1/For Iterator Subsystem/compute_next_step/If Action Subsystem1/For Iterator Subsystem/If Action Subsystem/If Action Subsystem3/phi_t/gradient_angle/ga_f ==
  data: x input; out output; y input; z input
function out = fcn(x, y, z)
out = zeros(1,3); 
out(1) = x;
out(2) = y;
out(3) = z;

== matlab function NDT_Localization/observation_callback/check_localizer/If Action Subsystem/register_measurement_impl/If Action Subsystem/If Action Subsystem/solve/If Action Subsystem1/For Iterator Subsystem/compute_next_step/If Action Subsystem1/For Iterator Subsystem/If Action Subsystem/If Action Subsystem3/phi_t/gradient_angle/ga_g ==
  data: x input; out output; y input; z input
function out = fcn(x, y, z)
out = zeros(1,3); 
out(1) = x;
out(2) = y;
out(3) = z;

== matlab function NDT_Localization/observation_callback/check_localizer/If Action Subsystem/register_measurement_impl/If Action Subsystem/If Action Subsystem/solve/set_jacobian ==
  data: jacobian output
function jacobian = fcn()

jacobian = zeros(6,1,"single");

== matlab function NDT_Localization/observation_callback/check_localizer/If Action Subsystem/register_measurement_impl/If Action Subsystem/If Action Subsystem/solve/If Action Subsystem1/For Iterator Subsystem/compute_next_step/If Action Subsystem1/For Iterator Subsystem/If Action Subsystem/If Action Subsystem3/phi_t/gradient_angle/ga_h ==
  data: x input; out output; y input; z input
function out = fcn(x, y, z)
out = zeros(1,3); 
out(1) = x;
out(2) = y;
out(3) = z;

== matlab function NDT_Localization/observation_callback/check_localizer/If Action Subsystem/register_measurement_impl/If Action Subsystem/If Action Subsystem/solve/If Action Subsystem1/For Iterator Subsystem/compute_next_step/If Action Subsystem1/For Iterator Subsystem/If Action Subsystem/If Action Subsystem3/phi_t/point_gradient ==
  data: hessian output; ga_a input; ga_b input; ga_c input; ga_d input; ga_e input; ga_f input; ga_g input; ga_h input
function hessian = fcn(ga_a, ga_b, ga_c, ga_d, ga_e, ga_f, ga_g, ga_h)

hessian = zeros(3,6,"single");
hessian(1,3) = ga_a;
hessian(2,3) = ga_b;
hessian(0,4) = ga_c;
hessian(1,4) = ga_d;
hessian(2,4) = ga_e;
hessian(0,5) = ga_f;
hessian(1,5) = ga_g;
hessian(2,5) = ga_h;

== matlab function NDT_Localization/observation_callback/check_localizer/If Action Subsystem/register_measurement_impl/If Action Subsystem/If Action Subsystem/solve/If Action Subsystem1/For Iterator Subsystem/compute_next_step/If Action Subsystem1/For Iterator Subsystem/If Action Subsystem/If Action Subsystem3/phi_t/set_jacobian ==
  data: jacobian output
function jacobian = fcn()

jacobian = zeros(6,1,"single");

== matlab function NDT_Localization/observation_callback/check_localizer/If Action Subsystem/register_measurement_impl/If Action Subsystem/If Action Subsystem/solve/If Action Subsystem1/For Iterator Subsystem/compute_next_step/If Action Subsystem1/For Iterator Subsystem/If Action Subsystem/If Action Subsystem3/psi_t/initial_objective_function/For Iterator Subsystem/Affine ==
  data: out output; u input
function out = fcn(u)

tform = affine3d;
pt = pointCloud(u);
xyz = pctransform(pt,tform);
out = xyz.Location;

== matlab function NDT_Localization/observation_callback/check_localizer/If Action Subsystem/register_measurement_impl/If Action Subsystem/If Action Subsystem/solve/If Action Subsystem1/For Iterator Subsystem/compute_next_step/If Action Subsystem1/For Iterator Subsystem/If Action Subsystem/If Action Subsystem3/psi_t/initial_objective_function/For Iterator Subsystem/MATLAB Function ==
  data: data input; pt output; index input
function pt = fcn(data,index)

pt = data(index);
